simulink model "Problem_3_Bilinear_Transformation"  (R2020b)
settings: Solver=VariableStepAuto  StartTime=0.0  StopTime=10.0  RelTol=1e-3
settings Model: Creator=Manoj  LastModifiedBy=Windows 10
settings DataIOCC: ExternalInput=[t, F]  SaveFormat=Structure

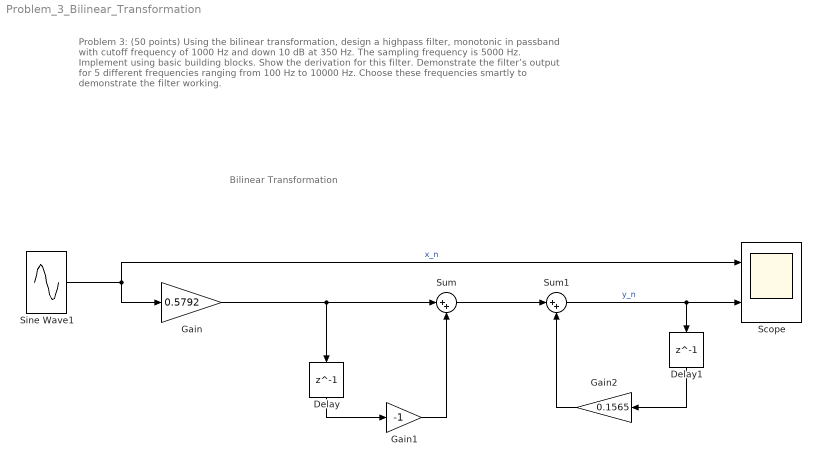
== system Problem_3_Bilinear_Transformation ==
  note: Bilinear Transformation
  note: Problem 3: (50 points) Using the bilinear transformation, design a highpass filter, monotonic in passband with cutoff frequency of 1000 Hz and down 10 dB at 350 Hz. The sampling frequency is 5000 Hz. Implement using basic building blocks. Show the derivation for this filter. Demonstrate the filter’s output for 5 different frequencies ranging from 100 Hz to 10000 Hz. Choose these frequencies smartly to demonstrate the filter working.
  Delay : Delay  DelayLength=1
  Delay1 : Delay  DelayLength=1
  Gain : Gain  Gain=0.5792
  Gain1 : Gain  Gain=-1
  Gain2 : Gain  Gain=0.1565
  Scope : Scope  NumInputPorts=2
  Sine Wave1 : Sin  Frequency=1000*6.28  SampleTime=2*10^-4
  Sum : Sum  Inputs=|++
  Sum1 : Sum  Inputs=|++
  wires:
  Sine Wave1/1 -> Gain/1, Scope/1  "x_n"
  Gain/1 -> Delay/1, Sum/1
  Delay/1 -> Gain1/1
  Gain1/1 -> Sum/2
  Sum/1 -> Sum1/1
  Sum1/1 -> Delay1/1, Scope/2  "y_n"
  Delay1/1 -> Gain2/1
  Gain2/1 -> Sum1/2
